simulink model "Robot_holonome_dynamique"  (R2023a)
settings: Solver=VariableStepAuto  StartTime=0.0  StopTime=10.0  RelTol=1e-3
settings Model: Creator=Administrateur  LastModifiedBy=Administrateur

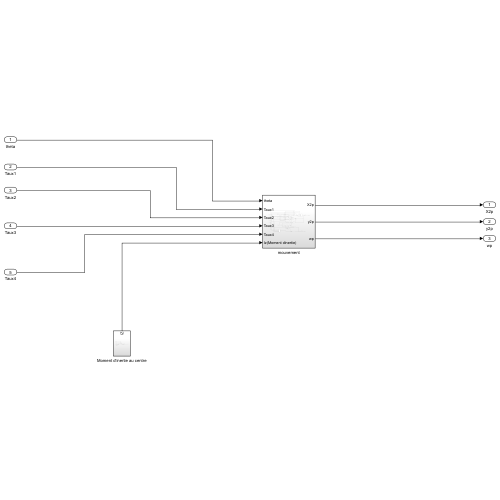
[thumbnail: Simulink's stored preview of the top-level diagram]
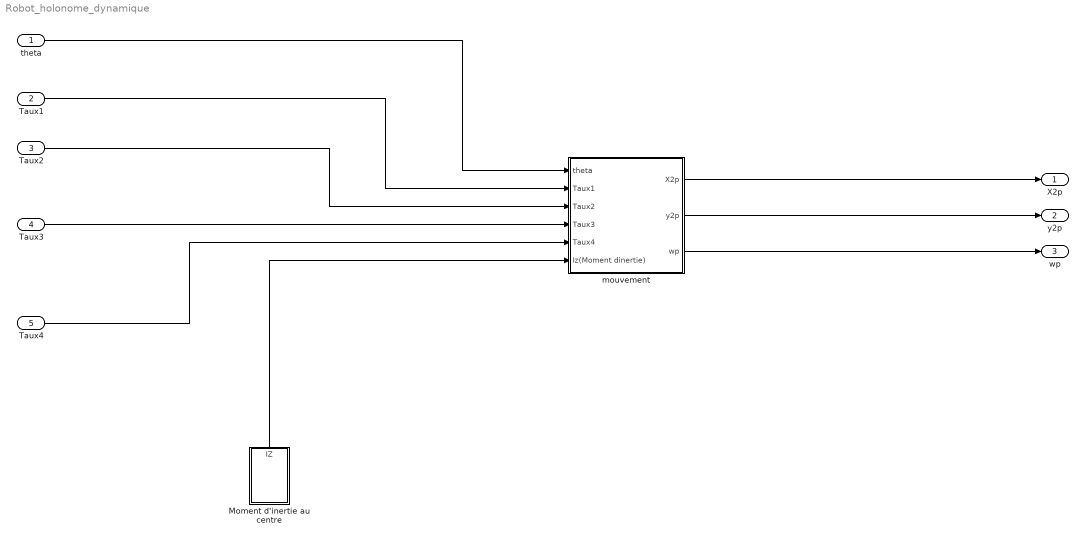
== system Robot_holonome_dynamique ==
  theta : Inport
  Taux1 : Inport  Port=2
  Taux2 : Inport  Port=3
  Taux3 : Inport  Port=4
  Taux4 : Inport  Port=5
  Moment d'inertie au centre : Subsystem
      settings: PortSchema="{\"entries\":[{\"content\":{\"sides\":[{\"content\":{},\"type\":\"ConnectorPlacement.EquallySpacedRectSide\",\"uuid\":\"7df1d69e-9fc5-49f7-ab14-2c6ab139a9b0\"},{\"content\":{\"side\":\"RIGHT\"},\"type\":\"ConnectorPlacement.EquallySpacedRectSide\",\"uuid\":\"ddcac711-cdc2-4f54-88b2-c084a0f547e4\"},{\"content\":{\"connectorIds\":[\"Out1\"],\"side\":\"TOP\"},\"type\":\"ConnectorPlacement.EquallySpacedRectSide\",\"uuid\":\"a5d37e4f-9664-4a43-9131-b5ab70e9787f\"}]},\"type\":\"ConnectorPlacement.EquallySpacedConnector\",\"uuid\":\"027eacd1-a6e4-46dc-8b7b-7d644007e566\"}],\"packageUris\":[\"http://schema.mathworks.com/mf0/Connector/R2020b\"],\"version\":\"1.0\"}"
  mouvement : Subsystem
  X2p : Outport
  y2p : Outport  Port=2
  wp : Outport  Port=3
  wires:
  theta/1 -> mouvement/1(theta)
  Taux1/1 -> mouvement/2(Taux1)
  Taux2/1 -> mouvement/3(Taux2)
  Taux3/1 -> mouvement/4(Taux3)
  Taux4/1 -> mouvement/5(Taux4)
  mouvement/1(X2p) -> X2p/1
  mouvement/2(y2p) -> y2p/1
  mouvement/3(wp) -> wp/1
  Moment d'inertie au centre/1(IZ) -> mouvement/6(Iz(Moment dinertie))

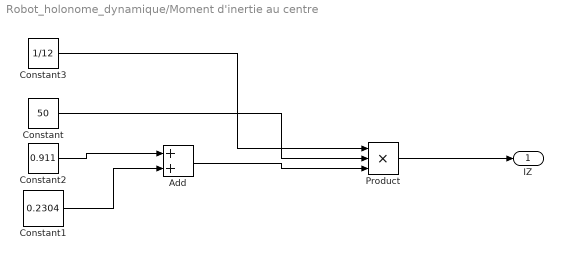
== system Robot_holonome_dynamique/Moment d'inertie au centre ==
  Add : Sum
  Constant : Constant  Value=50
  Constant1 : Constant  Value=0.2304
  Constant2 : Constant  Value=0.911
  Constant3 : Constant  Value=1/12
  Product : Product  Inputs=3
  IZ : Outport
  wires:
  Constant3/1 -> Product/1
  Add/1 -> Product/3
  Constant1/1 -> Add/2
  Constant/1 -> Product/2
  Product/1 -> IZ/1
  Constant2/1 -> Add/1

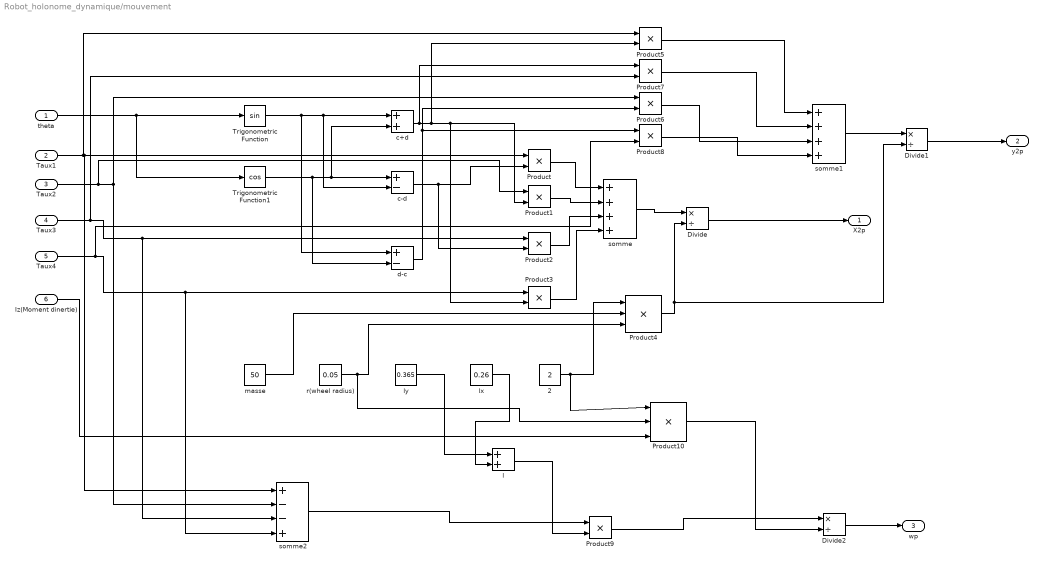
== system Robot_holonome_dynamique/mouvement ==
  theta : Inport
  Taux1 : Inport  Port=2
  Taux2 : Inport  Port=3
  Taux3 : Inport  Port=4
  Taux4 : Inport  Port=5
  Iz(Moment dinertie) : Inport  Port=6
  2 : Constant  Value=2
  Divide : Product  Inputs=*/
  Divide1 : Product  Inputs=*/
  Divide2 : Product  Inputs=*/
  Product{,1..3,5..9} (9 alike) : Product
  Product10 : Product  Inputs=3
  Product4 : Product  Inputs=3
  Trigonometric Function : Trigonometry
  Trigonometric Function1 : Trigonometry  Operator=cos
  c+d : Sum
  c-d : Sum  Inputs=+-
  d-c : Sum  Inputs=+-
  l : Sum
  lx : Constant  Value=0.26
  ly : Constant  Value=0.365
  masse : Constant  Value=50
  r(wheel radius) : Constant  Value=0.05
  somme : Sum  Inputs=++++
  somme1 : Sum  Inputs=++++
  somme2 : Sum  Inputs=+--+
  X2p : Outport
  y2p : Outport  Port=2
  wp : Outport  Port=3
  wires:
  2/1 -> Product10/1, Product4/1
  theta/1 -> Trigonometric Function1/1, Trigonometric Function/1
  Taux1/1 -> somme2/1, Product/1, Product5/1
  Product4/1 -> Divide1/2, Divide/2
  r(wheel radius)/1 -> Product10/2, Product4/3
  Taux2/1 -> somme2/2, Product6/1, Product1/1
  Iz(Moment dinertie)/1 -> Product10/3
  Taux3/1 -> Product7/2, somme2/3, Product2/1
  Product10/1 -> Divide2/2
  Product6/1 -> somme1/3
  Taux4/1 -> Product8/2, somme2/4, Product3/1
  c+d/1 -> Product7/1, Product5/2, Product3/2, Product1/2
  Divide1/1 -> y2p/1
  Trigonometric Function1/1 -> d-c/2, c-d/1, c+d/2
  somme/1 -> Divide/1
  Product5/1 -> somme1/1
  somme2/1 -> Product9/1
  somme1/1 -> Divide1/1
  l/1 -> Product9/2
  masse/1 -> Product4/2
  Product3/1 -> somme/4
  lx/1 -> l/2
  Product7/1 -> somme1/2
  Product8/1 -> somme1/4
  Product9/1 -> Divide2/1
  c-d/1 -> Product2/2, Product/2
  Trigonometric Function/1 -> d-c/1, c-d/2, c+d/1
  Divide/1 -> X2p/1
  Product1/1 -> somme/2
  d-c/1 -> Product8/1, Product6/2
  ly/1 -> l/1
  Divide2/1 -> wp/1
  Product2/1 -> somme/3
  Product/1 -> somme/1
